simulink model "robusto"  (R2021b)
settings: Solver=VariableStepAuto  StartTime=0.0  StopTime=10  RelTol=1e-3
values from neighbouring files (symbols this model uses):
  C = 2500*10^-6    (= 0.0025)    [paremetrosrobus.m]
  Em = 80    [paremetrosrobus.m]
  epsilon = 0.1    [paremetrosrobus.m]
  k1 = 90    [paremetrosrobus.m]
  k2 = 600    [paremetrosrobus.m]
  k3 = 600    [paremetrosrobus.m]
  L = 10*10^-3    (= 0.01)    [paremetrosrobus.m]
  R = 3    [paremetrosrobus.m]
  Rl = 45    [paremetrosrobus.m]
  w = 60    [paremetrosrobus.m]
  x2d = 0    [paremetrosrobus.m]
  x3d = 48    [paremetrosrobus.m]
settings Model: Creator=CIO  LastModifiedBy=LAPONE

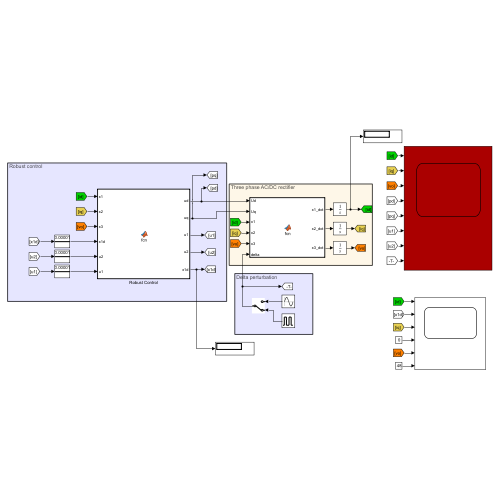
[thumbnail: Simulink's stored preview of the top-level diagram]
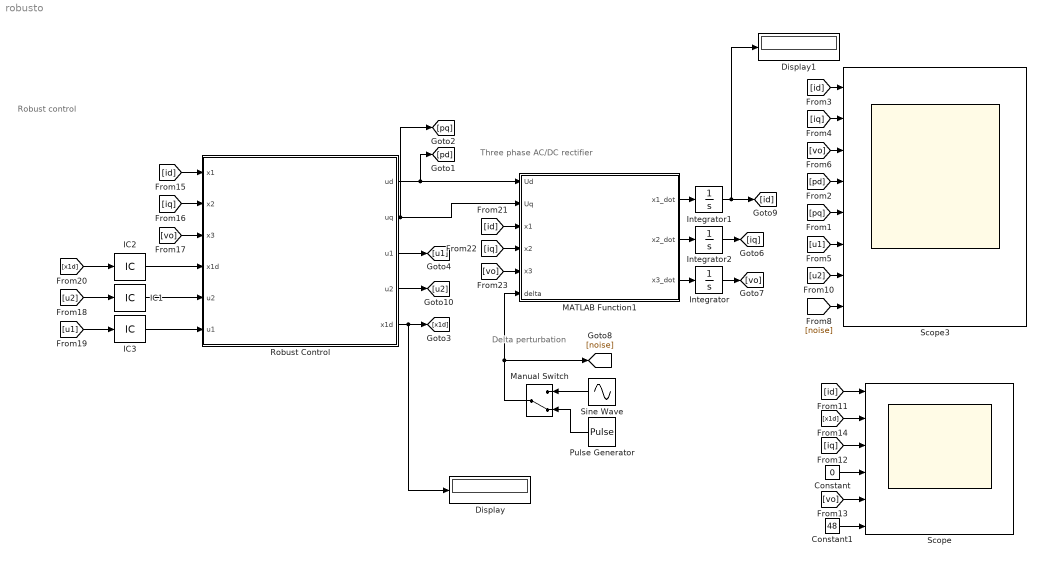
== system robusto ==
  note: Delta perturbation
  note: Three phase AC/DC rectifier
  note: Robust control
  Constant : Constant  Value=0
  Constant1 : Constant  Value=48
  Display : Display
  Display1 : Display
  IC1 : InitialCondition  Value=0.00001
  IC2 : InitialCondition  Value=0.00001
  IC3 : InitialCondition  Value=0.00001
  Integrator : Integrator  InitialCondition=0.1
  Integrator1 : Integrator  InitialCondition=0.1
  Integrator2 : Integrator  InitialCondition=0.1
  MATLAB Function1 : MATLAB Function  TreatAsAtomicUnit=on
  Manual Switch : ManualSwitch  CurrentSetting=0
  Pulse Generator : DiscretePulseGenerator  PulseType=Time based  Amplitude=50  Period=1  PulseWidth=20
  Robust Control : MATLAB Function  TreatAsAtomicUnit=on
  Scope : Scope  NumInputPorts=6
  Scope3 : Scope  NumInputPorts=8
  Sine Wave : Sin  Amplitude=10  Frequency=5  SampleTime=0
  wires:
  [id] -> Scope/1
  [x1d] -> Scope/2
  [iq] -> Scope/3
  Constant/1 -> Scope/4
  [vo] -> Scope/5
  Constant1/1 -> Scope/6
  [id] -> Robust Control/1(x1)
  [iq] -> Robust Control/2(x2)
  [vo] -> Robust Control/3(x3)
  IC2/1 -> Robust Control/4("x1d ")
  IC1/1 -> Robust Control/5("u2 ")
  IC3/1 -> Robust Control/6("u1 ")
  Robust Control/3(u1) -> [u1]
  Robust Control/4(u2) -> [u2]
  [u2] -> IC1/1
  [u1] -> IC3/1
  [x1d] -> IC2/1
  Sine Wave/1 -> Manual Switch/1
  Pulse Generator/1 -> Manual Switch/2
  Manual Switch/1 -> MATLAB Function1/6(delta), [noise]
  Robust Control/1(ud) -> [pd], MATLAB Function1/1(Ud)
  [id] -> MATLAB Function1/3(x1)
  [iq] -> MATLAB Function1/4(x2)
  [vo] -> MATLAB Function1/5(x3)
  MATLAB Function1/1(x1_dot) -> Integrator1/1
  MATLAB Function1/2(x2_dot) -> Integrator2/1
  MATLAB Function1/3(x3_dot) -> Integrator/1
  Integrator1/1 -> Display1/1, [id]
  Integrator2/1 -> [iq]
  Integrator/1 -> [vo]
  Robust Control/5(x1d) -> [x1d], Display/1
  Robust Control/2(uq) -> [pq], MATLAB Function1/2(Uq)
  [iq] -> Scope3/2
  [vo] -> Scope3/3
  [id] -> Scope3/1
  [pd] -> Scope3/4
  [pq] -> Scope3/5
  [u1] -> Scope3/6
  [u2] -> Scope3/7
  [noise] -> Scope3/8

== matlab function robusto/Robust Control ==
  data: x1 input; ud output; x2 input; x3 input; uq output; Em parameter; C parameter; L parameter; w parameter; R parameter; x3d parameter; x2d parameter; k3 parameter; k2 parameter; Rl parameter; u1 output; u2 output; x1d input; k1 parameter; x1d output; u2 input; u1 input; epsilon parameter
function [ud , uq, u1,u2,x1d] = fcn(x1, x2, x3,Em,C, L, w, R, x3d, x2d,k3, k2,Rl,x1d, k1,u2,u1,epsilon)

e1 = x1 - x1d; e2 = x2 - x2d;      e3 = x3 - x3d; 

%x1d = x1d_1;
x1d = (2*C*u2*(e3 + x3d))/(3*L*u1) - e1;
%x1d = -sqrt((2*(x3d)^2)/(3*L*Rl - (R/L) + (Em/L)));
%x1d = -(3^(1/2)*(Rl*(3*Rl*Em^2 - 8*R*x3d^2))^(1/2) + 3*Em*Rl)/(6*R*Rl);
 
%x1d = ((Em + 3*L^2 + (Em^2 + 6*Em*L^2 + 9*L^4 - 8*R*C*L*x3d^2)^(1/2))/(2*R));
%controls
%para evitar singularidades agregamos el termino epsilon donde corresponda


%uq = (2*L/(x3 + epsilon)) * ( -(R/L)*(e2 + x2d) + w*(e1 + x1d) + k2*sqrt(abs(e2))*sign(e2) );
 uq = (2*L/(x3 + epsilon)) * ( -(R/L)*(e2) + w*(e1 + x1d) + k2*sqrt(abs(e2))*sign(e2) );


u1 = ((-R/L)*(e1+x1d)) - (w*e2) + (Em/L) + (k1*sqrt(abs(e1))*sign(e1));
%u1 = ((-R/L)*(e1+x1d)) + (Em/L) + (k1*sqrt(abs(e1))*sign(e1));

%u2 = -(3/(4*C))*(e2 + x2d)*uq + (1/(Rl*C)) * (e3 + x3d) - k3*sqrt(abs(e3))*sign(e3);
%u2 = +(1/(Rl*C)) * (e3 + x3d) - k3*sqrt(abs(e3))*sign(e3);
u2 = -(3/(4*C))*(e2)*uq + (1/(Rl*C)) * (e3 + x3d) - k3*sqrt(abs(e3))*sign(e3);

ud =  ((4*C)/3) * u2/(x1 + epsilon) ;
%ud =  ((2*L)/1) * u1/(e3 + x3d + epsilon) ;

== matlab function robusto/MATLAB Function1 ==
  data: Ud input; Uq input; x1_dot output; x1 input; x2 input; x3 input; w parameter; L parameter; R parameter; Em parameter; delta input; x2_dot output; x3_dot output; C parameter; Rl parameter
function [x1_dot,x2_dot,x3_dot] = fcn(Ud,Uq,x1,x2,x3,w, L, R, Em, delta, C, Rl)

x1_dot = - ((R*x1)/(L)) - w*x2 - (x3*Ud)/(2*L) + (Em/L);
x2_dot = - R*x2/L + w*x1 - ((x3*Uq)/(2*L));
x3_dot = (3*x1*Ud)/(4*C) + (3*x2*Uq)/(4*C) - (((x3)/(Rl*C))+ delta) ;
